simulink model "Swing2D_01"  (R2018b)
settings: Solver=VariableStepAuto  StartTime=0.0  StopTime=10  RelTol=1e-3
InitFcn:
  | Swing2d_01_const
values from neighbouring files (symbols this model uses):
  d = 1    [Swing2d_01_const.m]
  g = 9.81    [Const_Vel_Est_02.m]    (also in Swing2d_01_const.m; constant_Rev01_4Agents_10.m; constant_Rev01_4Agents_9.m)
  I = 0.1    [Swing2d_01_const.m]
  k21 = 1    [Swing2d_01_const.m]
  k22 = 1    [Swing2d_01_const.m]
  m = 6    [Cons_AMFC_Quad_New_01.m]    (also in Const_Vel_Est_02.m; Swing2d_01_const.m = 1)
  vd = 10    [Swing2d_01_const.m]
settings Model: Creator=asafae  LastModifiedBy=asafae

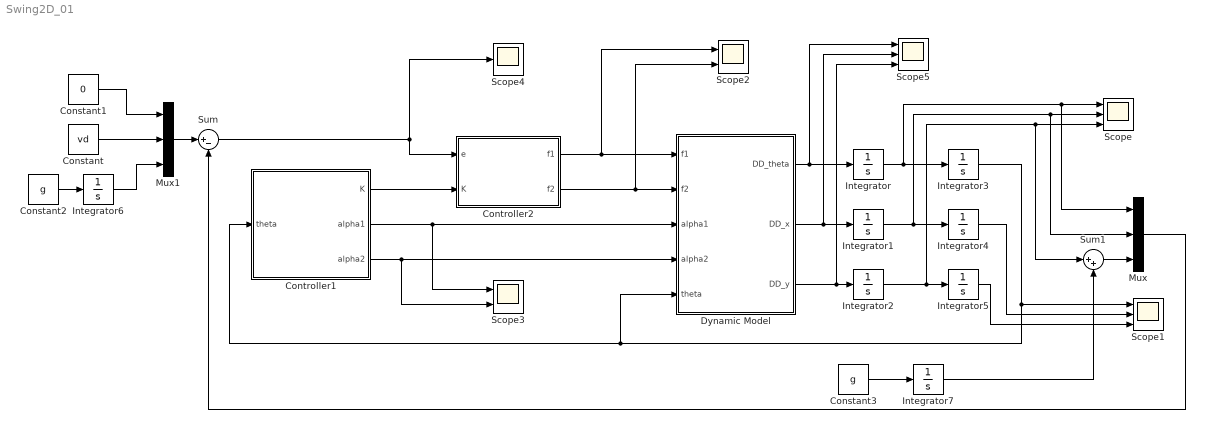
== system Swing2D_01 ==
  Constant : Constant  Value=vd
  Constant1 : Constant  Value=0
  Constant2 : Constant  Value=g
  Constant3 : Constant  Value=g
  Controller1 : MATLAB Function  TreatAsAtomicUnit=on
  Controller2 : MATLAB Function  TreatAsAtomicUnit=on
  Dynamic Model : MATLAB Function  TreatAsAtomicUnit=on
  Integrator{,1..2,4,6..7} (6 alike) : Integrator
  Integrator3 : Integrator  InitialCondition=1
  Integrator5 : Integrator  InitialCondition=10
  Mux : Mux  Inputs=3
  Mux1 : Mux  Inputs=3
  Scope : Scope  NumInputPorts=3
  Scope1 : Scope  NumInputPorts=3
  Scope2 : Scope  NumInputPorts=2
  Scope3 : Scope  NumInputPorts=2
  Scope4 : Scope
  Scope5 : Scope  NumInputPorts=3
  Sum : Sum  Inputs=|+-
  Sum1 : Sum  Inputs=|++
  wires:
  Controller1/2(alpha1) -> Dynamic Model/3(alpha1), Scope3/1
  Controller1/3(alpha2) -> Dynamic Model/4(alpha2), Scope3/2
  Controller1/1(K) -> Controller2/2(K)
  Controller2/2(f2) -> Dynamic Model/2(f2), Scope2/2
  Controller2/1(f1) -> Dynamic Model/1(f1), Scope2/1
  Dynamic Model/2(DD_x) -> Integrator1/1, Scope5/2
  Dynamic Model/3(DD_y) -> Scope5/3, Integrator2/1
  Integrator/1 -> Integrator3/1, Mux/1, Scope/1
  Integrator1/1 -> Integrator4/1, Mux/2, Scope/2
  Integrator2/1 -> Sum1/1, Scope/3, Integrator5/1
  Integrator3/1 -> Dynamic Model/5(theta), Controller1/1(theta), Scope1/1
  Integrator4/1 -> Scope1/2
  Integrator5/1 -> Scope1/3
  Sum/1 -> Scope4/1, Controller2/1(e)
  Mux1/1 -> Sum/1
  Constant/1 -> Mux1/2
  Constant1/1 -> Mux1/1
  Constant2/1 -> Integrator6/1
  Constant3/1 -> Integrator7/1
  Integrator7/1 -> Sum1/2
  Sum1/1 -> Mux/3
  Mux/1 -> Sum/2
  Integrator6/1 -> Mux1/3
  Dynamic Model/1(DD_theta) -> Integrator/1, Scope5/1

== matlab function Swing2D_01/Controller1 ==
  data: theta input; K output; alpha1 output; alpha2 output; k21 parameter; k22 parameter; d parameter; m parameter; I parameter
function [K,alpha1,alpha2] = fcn(theta,k21, k22,d, m, I)

k31 = 1;
k32 = 1;

K1 = k21 / k31;
K2 = k22 / k32;

alpha1 = atan( (-K1*sin(theta) + cos(theta)) / (K1*cos(theta) + sin(theta)) );
alpha2 = atan( (-K2*sin(theta) + cos(theta)) / (K2*cos(theta) + sin(theta)) );

k11 = (d * m / I) * k31 * (-K1*sin(theta) + cos(theta));
k12 = -(d * m / I) * k32 * (-K2*sin(theta) + cos(theta));

K = [k11 k12;k21 k22;k31 k32];

end

== matlab function Swing2D_01/Dynamic Model ==
  data: f1 input; DD_theta output; f2 input; alpha1 input; alpha2 input; theta input; DD_x output; DD_y output; d parameter; I parameter; m parameter; g parameter
function [DD_theta,DD_x,DD_y] = fcn(f1,f2,alpha1,alpha2,theta,d, I, m, g)

DD_theta = (d/I) * ( (f1 * sin(alpha1)) - (f2 * sin(alpha2)) );
DD_x = (1/m) * ( (f1 * cos(alpha1 + theta)) + (f2 * cos(alpha2 + theta)) );
DD_y = -g + (1/m) * ( (f1 * sin(alpha1 + theta)) + (f2 * sin(alpha2 + theta)) );

end

== matlab function Swing2D_01/Controller2 ==
  data: e input; f1 output; K input; xd_dd_M parameter; f2 output
function [f1,f2] = fcn(e,K,xd_dd_M)

SGN = zeros(3);
SGN(1,1) = sign(e(1));
SGN(2,2) = sign(e(2));
SGN(3,3) = sign(e(3));

F = ( (K'*K)^(-1) * K' ) * SGN * xd_dd_M;
f1 = F(1);
f2 = F(2);

end
